simulink model "Lazoabierto"  (R2023a)
settings: Solver=ode15s  StartTime=0.0  StopTime=10.0  MaxStep=1e-5  RelTol=1e-6
settings Model: Creator=jesus  LastModifiedBy=jesus
settings DataIOCC: ReturnWorkspaceOutputs=off  TimeSaveName=t
settings DebuggingCC: AlgebraicLoopMsg=none  ArtificialAlgebraicLoopMsg=none  BlockPriorityViolationMsg=error  MaxConsecutiveZCsMsg=none  ModelReferenceExtraNoncontSigs=none  OperatingPointInterfaceChecksumMismatchMsg=none

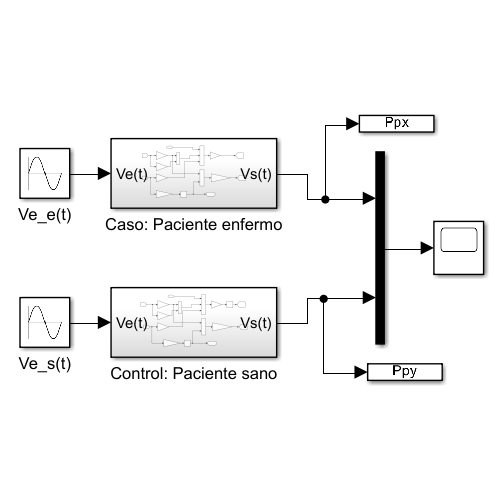
[thumbnail: Simulink's stored preview of the top-level diagram]
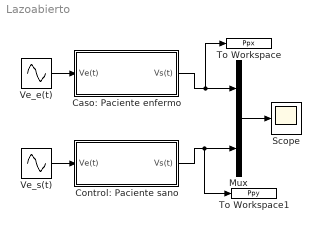
== system Lazoabierto ==
  Caso: Paciente enfermo : Subsystem
  Control: Paciente sano : Subsystem
  Mux : Mux  Inputs=2
  Scope : Scope
  To Workspace : ToWorkspace  VariableName=Ppx  SampleTime=-1
  To Workspace1 : ToWorkspace  VariableName=Ppy  SampleTime=-1
  Ve_e(t) : Sin  Amplitude=0.4  Frequency=2*pi  SampleTime=0
  Ve_s(t) : Sin  Frequency=2*pi  SampleTime=0
  wires:
  Mux/1 -> Scope/1
  Caso: Paciente enfermo/1(Vs(t)) -> To Workspace/1, Mux/1
  Control: Paciente sano/1(Vs(t)) -> To Workspace1/1, Mux/2
  Ve_e(t)/1 -> Caso: Paciente enfermo/1(Ve(t))
  Ve_s(t)/1 -> Control: Paciente sano/1(Ve(t))

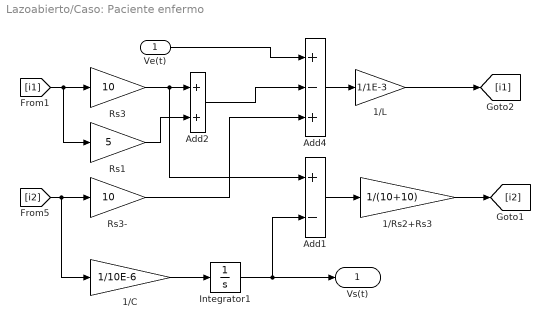
== system Lazoabierto/Caso: Paciente enfermo ==
  Ve(t) : Inport
  1/C : Gain  Gain=1/10E-6
  1/L : Gain  Gain=1/1E-3
  1/Rs2+Rs3 : Gain  Gain=1/(10+10)
  Add1 : Sum  Inputs=+-
  Add2 : Sum
  Add4 : Sum  Inputs=+-+
  Integrator1 : Integrator
  Rs1 : Gain  Gain=5
  Rs3 : Gain  Gain=10
  Rs3- : Gain  Gain=10
  Vs(t) : Outport
  wires:
  Add1/1 -> 1/Rs2+Rs3/1
  Rs1/1 -> Add2/2
  [i2] -> 1/C/1, Rs3-/1
  [i1] -> Rs1/1, Rs3/1
  1/Rs2+Rs3/1 -> [i2]
  Ve(t)/1 -> Add4/1
  Rs3/1 -> Add2/1, Add1/1
  Add4/1 -> 1/L/1
  1/C/1 -> Integrator1/1
  Add2/1 -> Add4/2
  Rs3-/1 -> Add4/3
  Integrator1/1 -> Vs(t)/1, Add1/2
  1/L/1 -> [i1]

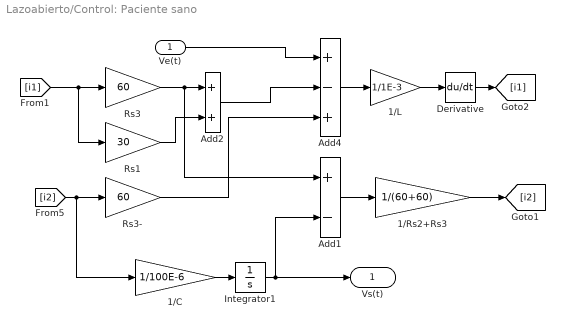
== system Lazoabierto/Control: Paciente sano ==
  Ve(t) : Inport
  1/C : Gain  Gain=1/100E-6
  1/L : Gain  Gain=1/1E-3
  1/Rs2+Rs3 : Gain  Gain=1/(60+60)
  Add1 : Sum  Inputs=+-
  Add2 : Sum
  Add4 : Sum  Inputs=+-+
  Derivative : Derivative
  Integrator1 : Integrator
  Rs1 : Gain  Gain=30
  Rs3 : Gain  Gain=60
  Rs3- : Gain  Gain=60
  Vs(t) : Outport
  wires:
  Ve(t)/1 -> Add4/1
  Add4/1 -> 1/L/1
  [i1] -> Rs1/1, Rs3/1
  [i2] -> 1/C/1, Rs3-/1
  Rs3/1 -> Add2/1, Add1/1
  Rs1/1 -> Add2/2
  Add2/1 -> Add4/2
  Rs3-/1 -> Add4/3
  1/L/1 -> Derivative/1
  1/Rs2+Rs3/1 -> [i2]
  1/C/1 -> Integrator1/1
  Integrator1/1 -> Add1/2, Vs(t)/1
  Add1/1 -> 1/Rs2+Rs3/1
  Derivative/1 -> [i1]
